simulink subsystem "Part1"  (R2024b)
settings: Solver=VariableStepAuto  StartTime=0.0  StopTime=10.0  RelTol=1e-3
libraries: simulink x6, ctrlSharedLib x2, sharedTrackingLibrary x1
settings Model: Creator=av200  LastModifiedBy=av200

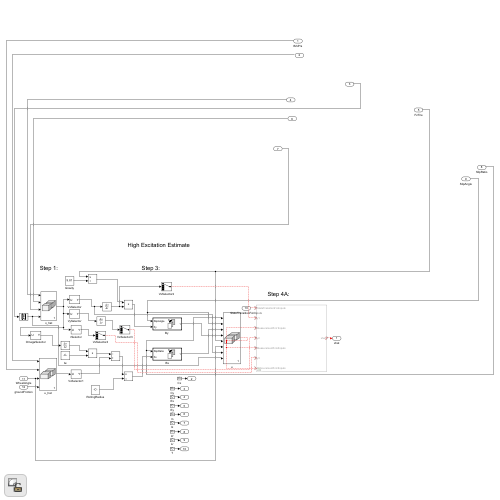
[thumbnail: Simulink's stored preview of the top-level diagram]
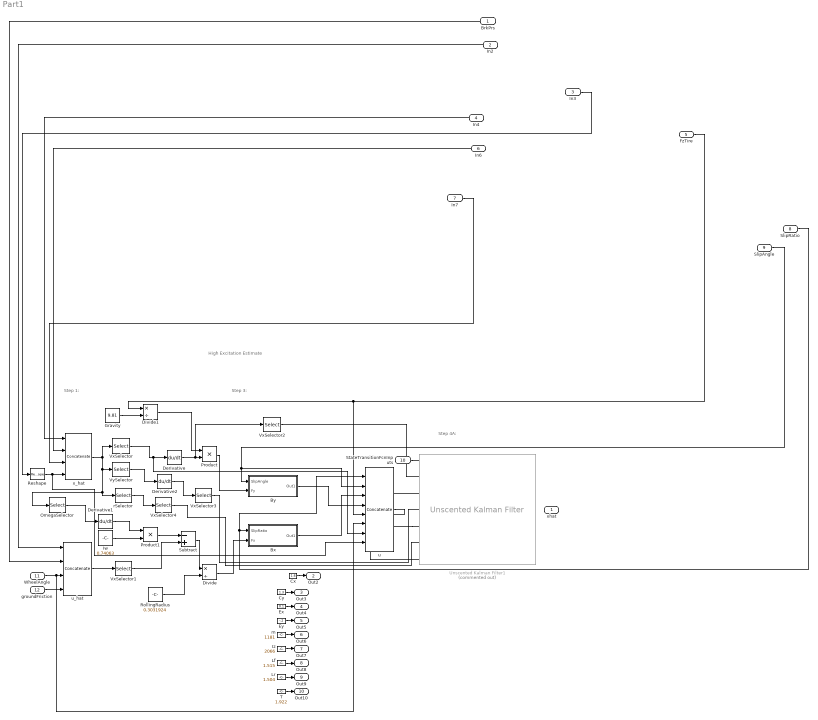
== system Part1 ==
  note: Step 3:
  note: Step 1:
  note: Step 4A:
  note: High Excitation Estimate
  BrkPrs : Inport
  In2 : Inport  Port=2
  In3 : Inport  Port=3
  In4 : Inport  Port=4
  FzTire : Inport  Port=5
  In6 : Inport  Port=6
  In7 : Inport  Port=7
  SlipRatio : Inport  Port=8
  SlipAngle : Inport  Port=9
  StateTransitionFcnInputs : Inport  Port=10
  WheelAngle : Inport  Port=11
  groundFriction : Inport  Port=12
  Bx : Subsystem  TreatAsAtomicUnit=on
  "By " : Subsystem  TreatAsAtomicUnit=on
  Cx : Constant  Value=1.6
  Cy : Constant  Value=1.3
  Derivative : Derivative
  Derivative1 : Derivative
  Derivative2 : Derivative
  Divide : Product  Inputs=*/
  Divide1 : Product  Inputs=*/
  Ex : Constant  Value=0.1
  Ey : Constant  Value=-.2
  Gravity : Constant  Value=9.81
  Iw : Constant  Value=0.74063
  Iz : Constant  Value=2066
  Lf : Constant  Value=1.515
  Lr : Constant  Value=1.504
  OmegaSelector : Selector  InputPortWidth=16  IndexOptions=Index vector (dialog)  Indices=13:16  OutputSizes=1
  Product : Product
  Product1 : Product
  Reshape : Reshape  OutputDimensionality=Column vector (2-D)
  RollingRadius : Constant  Value=0.3031924
  Subtract : Sum  Inputs=-+
  T : Constant  Value=1.922
  Unscented Kalman Filter1 : sharedTrackingLibrary/Unscented Kalman Filter  Commented=on  StateTransitionFcn=myStateTransitionFcn  HasAdditiveProcessNoise=Additive  ProcessNoise=eye(4) * 0.1  HasTimeVaryingProcessNoise=off  HasStateTransitionFcnExtraArgument=1  InitialState=[0.8; 0.8; 0.8; 0.8]  InitialStateCovariance=1  Alpha=1e-3  Beta=2  Kappa=0  MeasurementFcn1=myMeasAx  HasMeasurementEnablePort1=off  HasAdditiveMeasurementNoise1=Additive  MeasurementNoise1=1e-2  HasTimeVaryingMeasurementNoise1=off  HasMeasurementFcnExtraArgument1=1  HasMeasurementWrapping1=off  MeasurementFcn2=myMeasAy  HasMeasurementEnablePort2=off  HasAdditiveMeasurementNoise2=Additive  MeasurementNoise2=1e-2  HasTimeVaryingMeasurementNoise2=off  HasMeasurementFcnExtraArgument2=1  HasMeasurementWrapping2=off  MeasurementFcn3=myMeasR  HasMeasurementEnablePort3=off  HasAdditiveMeasurementNoise3=Additive  MeasurementNoise3=1e-2  HasTimeVaryingMeasurementNoise3=off  HasMeasurementFcnExtraArgument3=1  HasMeasurementWrapping3=off  MeasurementFcn4=myMeasurementFcn  HasMeasurementEnablePort4=off  HasAdditiveMeasurementNoise4=Additive  MeasurementNoise4=1  HasTimeVaryingMeasurementNoise4=off  HasMeasurementFcnExtraArgument4=0  HasMeasurementWrapping4=off  MeasurementFcn5=myMeasurementFcn  HasMeasurementEnablePort5=off  HasAdditiveMeasurementNoise5=Additive  MeasurementNoise5=1  HasTimeVaryingMeasurementNoise5=off  HasMeasurementFcnExtraArgument5=0  HasMeasurementWrapping5=off  EnableMultirate=off  StateTransitionFcnSampleTime=1  MeasurementFcn1SampleTime=1  MeasurementFcn2SampleTime=1  MeasurementFcn3SampleTime=1  MeasurementFcn4SampleTime=1  MeasurementFcn5SampleTime=1  UseCurrentEstimator=on  OutputStateCovariance=off  DataType=double  SampleTime=0.001  NumberOfMeasurements=3
      settings: LibrarySourceBlock=cstblocks/State Estimation/Unscented Kalman Filter
  VxSelector : Selector  InputPortWidth=16  IndexOptions=Index vector (dialog)  Indices=5:8  OutputSizes=1
  VxSelector1 : Selector  InputPortWidth=16  IndexOptions=Index vector (dialog)  Indices=1:4  OutputSizes=1
  VxSelector2 : Selector  InputPortWidth=4  IndexOptions=Index vector (dialog)  Indices=1:1  OutputSizes=1
  VxSelector3 : Selector  InputPortWidth=4  IndexOptions=Index vector (dialog)  Indices=1:1  OutputSizes=1
  VxSelector4 : Selector  InputPortWidth=4  IndexOptions=Index vector (dialog)  Indices=1:1  OutputSizes=1
  VySelector : Selector  InputPortWidth=16  IndexOptions=Index vector (dialog)  Indices=5:8  OutputSizes=1
  m : Constant  Value=1181
  rSelector : Selector  InputPortWidth=16  IndexOptions=Index vector (dialog)  Indices=9:12  OutputSizes=1
  u : Concatenate  NumInputs=8  Mode=Multidimensional array
  u_hat : Concatenate  NumInputs=4  Mode=Multidimensional array
  x_hat : Concatenate  NumInputs=4  Mode=Multidimensional array
  xhat : Outport
  Out2 : Outport  Port=2
  Out3 : Outport  Port=3
  Out4 : Outport  Port=4
  Out5 : Outport  Port=5
  Out6 : Outport  Port=6
  Out7 : Outport  Port=7
  Out8 : Outport  Port=8
  Out9 : Outport  Port=9
  Out10 : Outport  Port=10
  wires:
  Iw/1 -> Product1/2
  VxSelector1/1 -> Subtract/2
  Product/1 -> "By "/2(Fy)
  u/1 -> ?
  Reshape/1 -> x_hat/4, u/8
  FzTire/1 -> u/5, Divide1/1
  Lf/1 -> Out8/1
  RollingRadius/1 -> Divide/2
  VySelector/1 -> Derivative2/1
  Product1/1 -> Subtract/1
  m/1 -> Out6/1
  VxSelector/1 -> Derivative/1, u/7
  Divide/1 -> Bx/2(Fx)
  Bx/1(Out1) -> u/3
  x_hat/1 -> OmegaSelector/1, rSelector/1, VySelector/1, VxSelector/1
  u_hat/1 -> VxSelector1/1
  In7/1 -> x_hat/3
  Divide1/1 -> Product/1
  T/1 -> Out10/1
  In3/1 -> Reshape/1
  WheelAngle/1 -> u_hat/3, u/6
  Gravity/1 -> Divide1/2
  groundFriction/1 -> u_hat/4
  SlipAngle/1 -> u/2, "By "/1(SlipAngle)
  Derivative2/1 -> VxSelector3/1
  StateTransitionFcnInputs/1 -> ?
  Lr/1 -> Out9/1
  ? -> xhat/1
  Subtract/1 -> Divide/1
  SlipRatio/1 -> Bx/1(SlipRatio), u/1
  "By "/1(Out1) -> u/4
  OmegaSelector/1 -> Derivative1/1
  Ey/1 -> Out5/1
  rSelector/1 -> VxSelector4/1
  Derivative1/1 -> Product1/1
  Iz/1 -> Out7/1
  VxSelector2/1 -> ?
  BrkPrs/1 -> u_hat/2
  VxSelector4/1 -> ?
  Derivative/1 -> Product/2, VxSelector2/1
  VxSelector3/1 -> ?
  Cx/1 -> Out2/1
  In2/1 -> u_hat/1
  In4/1 -> x_hat/1
  In6/1 -> x_hat/2
  Cy/1 -> Out3/1
  Ex/1 -> Out4/1

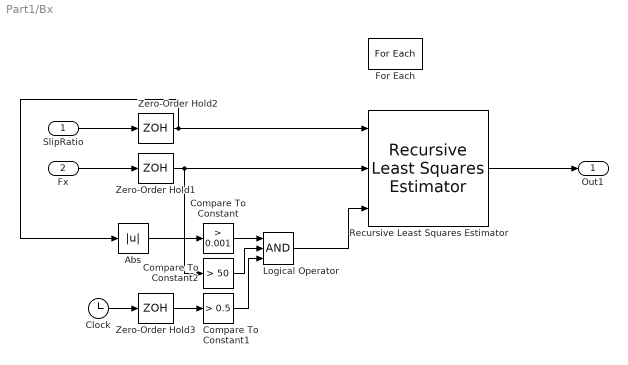
== system Part1/Bx ==
  SlipRatio : Inport  Partition=on  PartitionDimension=1  PartitionWidth=1  PartitionOffset=0
  Fx : Inport  Port=2  Partition=on  PartitionDimension=1  PartitionWidth=1  PartitionOffset=0
  Abs : Abs  SaturateOnIntegerOverflow=off
  Clock : Clock
  Compare To Constant : simulink/Logic and Bit Operations/Compare To Constant  relop=>  const=0.001  OutDataTypeStr=boolean
  Compare To Constant1 : simulink/Logic and Bit Operations/Compare To Constant  relop=>  const=0.5  OutDataTypeStr=boolean
  Compare To Constant2 : simulink/Logic and Bit Operations/Compare To Constant  relop=>  const=50  OutDataTypeStr=boolean
  For Each : ForEach  DisableCoverage=on
  Logical Operator : Logic  Inputs=3  AllPortsSameDT=off  OutDataTypeStr=boolean
  Recursive Least Squares Estimator : ctrlSharedLib/Recursive Least Squares Estimator  InitialEstimateSource=Internal  InitialParameterData=1e5  P0=1e5  InitialRegressors=0  InitialOutputs=0  History=Infinite  WindowLength=200  EstimationMethod=Forgetting Factor  AdaptationParameter=0.995  HasTimeVaryingAdaptationParameter=off  NormalizationBias=eps  OutputError=off  OutputP=off  AddEnablePort=on  InputProcessing=Sample-based  Ts=-1
  Zero-Order Hold1 : ZeroOrderHold  SampleTime=0.001
  Zero-Order Hold2 : ZeroOrderHold  SampleTime=0.001
  Zero-Order Hold3 : ZeroOrderHold  SampleTime=0.001
  Out1 : Outport  ConcatenationDimension=1
  wires:
  Compare To Constant2/1 -> Logical Operator/2
  Zero-Order Hold3/1 -> Compare To Constant1/1
  Logical Operator/1 -> Recursive Least Squares Estimator/3
  Compare To Constant1/1 -> Logical Operator/3
  Clock/1 -> Zero-Order Hold3/1
  Abs/1 -> Compare To Constant/1
  Compare To Constant/1 -> Logical Operator/1
  Zero-Order Hold1/1 -> Recursive Least Squares Estimator/2, Compare To Constant2/1
  Zero-Order Hold2/1 -> Recursive Least Squares Estimator/1, Abs/1
  Recursive Least Squares Estimator/1 -> Out1/1
  Fx/1 -> Zero-Order Hold1/1
  SlipRatio/1 -> Zero-Order Hold2/1

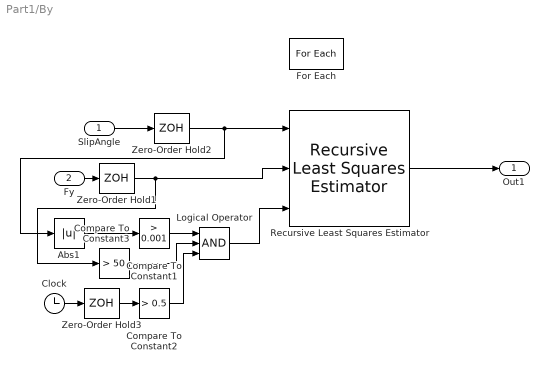
== system Part1/By  ==
  SlipAngle : Inport  Partition=on  PartitionDimension=1  PartitionWidth=1  PartitionOffset=0
  Fy : Inport  Port=2  Partition=on  PartitionDimension=1  PartitionWidth=1  PartitionOffset=0
  Abs1 : Abs  SaturateOnIntegerOverflow=off
  Clock : Clock
  Compare To Constant1 : simulink/Logic and Bit Operations/Compare To Constant  relop=>  const=0.001  OutDataTypeStr=boolean
  Compare To Constant2 : simulink/Logic and Bit Operations/Compare To Constant  relop=>  const=0.5  OutDataTypeStr=boolean
  Compare To Constant3 : simulink/Logic and Bit Operations/Compare To Constant  relop=>  const=50  OutDataTypeStr=boolean
  For Each : ForEach  DisableCoverage=on
  Logical Operator : Logic  Inputs=3  AllPortsSameDT=off  OutDataTypeStr=boolean
  Recursive Least Squares Estimator : ctrlSharedLib/Recursive Least Squares Estimator  InitialEstimateSource=Internal  InitialParameterData=1e5  P0=1e5  InitialRegressors=0  InitialOutputs=0  History=Infinite  WindowLength=200  EstimationMethod=Forgetting Factor  AdaptationParameter=0.995  HasTimeVaryingAdaptationParameter=off  NormalizationBias=eps  OutputError=off  OutputP=off  AddEnablePort=on  InputProcessing=Sample-based  Ts=-1
  Zero-Order Hold1 : ZeroOrderHold  SampleTime=0.001
  Zero-Order Hold2 : ZeroOrderHold  SampleTime=0.001
  Zero-Order Hold3 : ZeroOrderHold  SampleTime=0.001
  Out1 : Outport  ConcatenationDimension=1
  wires:
  Compare To Constant3/1 -> Logical Operator/2
  Zero-Order Hold3/1 -> Compare To Constant2/1
  Clock/1 -> Zero-Order Hold3/1
  Logical Operator/1 -> Recursive Least Squares Estimator/3
  Compare To Constant2/1 -> Logical Operator/3
  Abs1/1 -> Compare To Constant1/1
  Compare To Constant1/1 -> Logical Operator/1
  Zero-Order Hold1/1 -> Recursive Least Squares Estimator/2, Compare To Constant3/1
  Zero-Order Hold2/1 -> Recursive Least Squares Estimator/1, Abs1/1
  Recursive Least Squares Estimator/1 -> Out1/1
  Fy/1 -> Zero-Order Hold1/1
  SlipAngle/1 -> Zero-Order Hold2/1
